simulink model "revLimModelTester"  (R2017a)
settings: Solver=FixedStepDiscrete  StartTime=0.0  StopTime=3  FixedStep=0.001  RelTol=1e-3  EnableMultiTasking=on
libraries: simulink x1
settings Model: Creator=Johnny ZWall  LastModifiedBy=Johnny ZWall
settings DataIOCC: LimitDataPoints=on
settings OptimizationCC: UseDivisionForNetSlopeComputation=on  UseFloatMulNetSlope=on  DefaultUnderspecifiedDataType=single  UseSpecifiedMinMax=on  EnhancedBackFolding=on  BooleansAsBitfields=on  PassReuseOutputArgsAs=Individual arguments  StateBitsets=on  DataBitsets=on  ZeroExternalMemoryAtStartup=off  ZeroInternalMemoryAtStartup=off  NoFixptDivByZeroProtection=on  EfficientFloat2IntCast=on  OptimizeBlockOrder=speed
settings DebuggingCC: ParameterTunabilityLossMsg=error  AllowSymbolicDim=off  SFUnexpectedBacktrackingDiag=warning  SFNoUnconditionalDefaultTransitionDiag=warning  SFExecutionAtInitializationDiag=none
settings HardwareCC: ProdBitPerInt=16  ProdBitPerPointer=16  ProdBitPerSizeT=16  ProdBitPerPtrDiffT=16  ProdLargestAtomicFloat=None  ProdWordSize=8  ProdHWDeviceType=Atmel->AVR
settings ModelReferenceCC: PropagateSignalLabelsOutOfModel=off
settings SFSimCC: MATLABDynamicMemAlloc=off
settings RTWCC: SystemTargetFile=realtime.tlc  GenCodeOnly=on  GenerateMakefile=off  TemplateMakefile=realtime.tmf  Description=Run on Target Hardware  GenerateReport=on  RTWVerbose=off  BuildConfiguration=Faster Runs  IncludeHyperlinkInReport=on  LaunchReport=on  GenerateTraceInfo=on  GenerateTraceReport=on  GenerateTraceReportSl=on  GenerateTraceReportSf=on  GenerateTraceReportEml=on  CheckMdlBeforeBuild=Warning
settings CodeAppCC: ForceParamTrailComments=on  IgnoreCustomStorageClasses=off  OperatorAnnotations=on  SimulinkDataObjDesc=on  SFDataObjDesc=on  MATLABFcnDesc=on  CustomSymbolStrGlobalVar=rt$N$M  CustomSymbolStrType=$N$M  CustomSymbolStrFcn=$N$M$F  CustomSymbolStrMacro=$N$M  DefineNamingRule=LowerCase  ParamNamingRule=UpperCase  SignalNamingRule=LowerCase  InsertBlockDesc=on  MATLABSourceComments=on  InternalIdentifier=Classic
settings STFCustomTargetCC: TargetLibSuffix=.a  MultiwordLength=256  GenerateSampleERTMain=on  CombineOutputUpdateFcns=on  ERTCustomFileBanners=on  SupportContinuousTime=off  SupportNonInlinedSFcns=off  RemoveResetFunc=on  MATLABClassNameForMDSCustomization=Simulink.SoftwareTarget.ERTCustomization  GRTInterface=off  SystemTargetFile=realtime.tlc
settings ERTTargetCC: GenerateSampleERTMain=on  ParMdlRefBuildCompliant=off  CompOptLevelCompliant=off  ConcurrentExecutionCompliant=off  ERTFirstTimeCompliant=off  ModelStepFunctionPrototypeControlCompliant=off  CPPClassGenCompliant=off  UseToolchainInfoCompliant=off  ERTCustomFileTemplate=realtime_file_process.tlc
settings ConfigComp: CovMetricSettings=dw  CovHtmlReporting=on  CovSaveCumulativeToWorkspaceVar=on  CovSaveSingleToWorkspaceVar=on  CovExternalEMLEnable=off

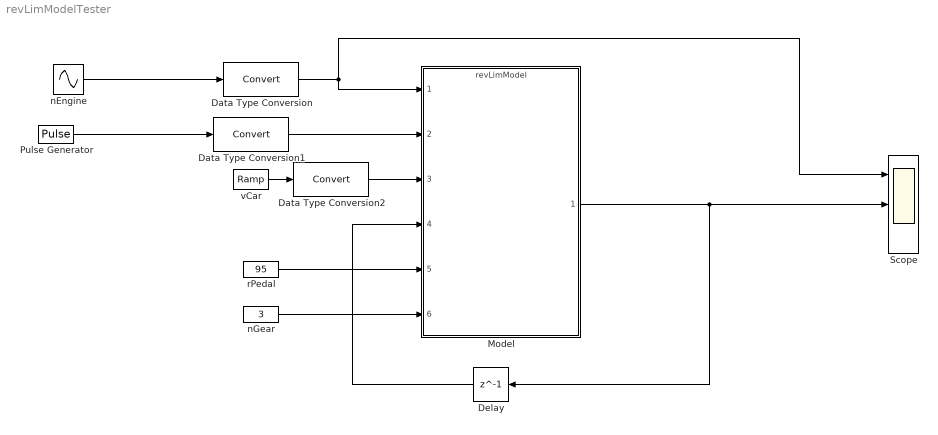
== system revLimModelTester ==
  Data Type Conversion : DataTypeConversion
  Data Type Conversion1 : DataTypeConversion
  Data Type Conversion2 : DataTypeConversion
  Delay : Delay  DelayLength=1  InitialCondition=0
  Model : ModelReference  ModelNameDialog=revLimModel.slx  SimulationMode=Normal  ModelReferenceVersion=1.106
  Pulse Generator : DiscretePulseGenerator  PulseType=Time based  Period=10  PulseWidth=50  PhaseDelay=.2
  Scope : Scope  NumInputPorts=3
  nEngine : Sin  Amplitude=1200  Bias=4000  Frequency=6  SampleTime=0
  nGear : Constant  Value=3  OutDataTypeStr=uint8
  rPedal : Constant  Value=95  OutDataTypeStr=single
  vCar : simulink/Sources/Ramp  slope=5  start=0  X0=44
  wires:
  Pulse Generator/1 -> Data Type Conversion1/1
  Model/1 -> Scope/2, Delay/1
  vCar/1 -> Data Type Conversion2/1
  Delay/1 -> Model/4
  rPedal/1 -> Model/5
  nGear/1 -> Model/6
  Data Type Conversion/1 -> Model/1, Scope/1
  Data Type Conversion1/1 -> Model/2
  Data Type Conversion2/1 -> Model/3
  nEngine/1 -> Data Type Conversion/1
